simulink subsystem "OpcodeDecoder"  (R2024b)
settings: Solver=VariableStepAuto  StartTime=0.0  StopTime=10.0  RelTol=1e-3
settings Model: Creator=stefano  LastModifiedBy=stefano

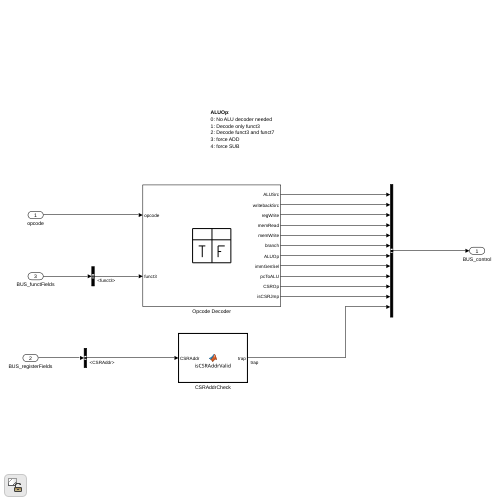
[thumbnail: Simulink's stored preview of the top-level diagram]
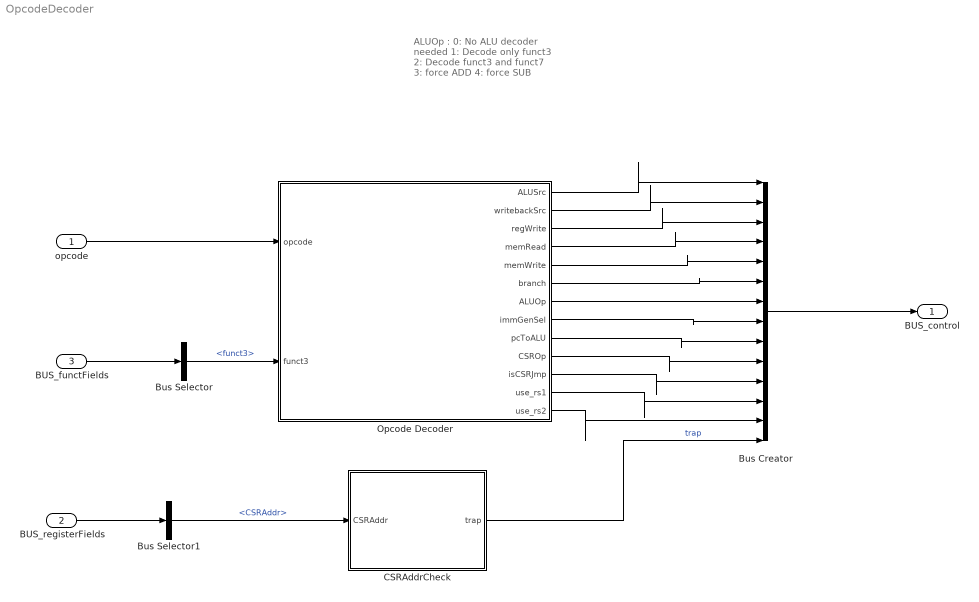
== system OpcodeDecoder ==
  note: ALUOp :
      | 0: No ALU decoder needed
      | 1: Decode only funct3
      | 2: Decode funct3 and funct7
      | 3: force ADD
      | 4: force SUB
  opcode : Inport
  BUS_registerFields : Inport  Port=2
  BUS_functFields : Inport  Port=3
  Bus Creator : BusCreator  Inputs=14
  Bus Selector : BusSelector  OutputSignals=funct3
  Bus Selector1 : BusSelector  OutputSignals=CSRAddr
  CSRAddrCheck : MATLAB Function  TreatAsAtomicUnit=on
  Opcode Decoder : Truth Table  TreatAsAtomicUnit=on
  BUS_control : Outport
  wires:
  Opcode Decoder/5(memWrite) -> Bus Creator/5
  opcode/1 -> Opcode Decoder/1(opcode)
  Opcode Decoder/8(immGenSel) -> Bus Creator/8
  Opcode Decoder/4(memRead) -> Bus Creator/4
  Opcode Decoder/2(writebackSrc) -> Bus Creator/2
  Opcode Decoder/3(regWrite) -> Bus Creator/3
  Bus Creator/1 -> BUS_control/1
  Opcode Decoder/1(ALUSrc) -> Bus Creator/1
  Opcode Decoder/7(ALUOp) -> Bus Creator/7
  Opcode Decoder/9(pcToALU) -> Bus Creator/9
  Opcode Decoder/6(branch) -> Bus Creator/6
  BUS_functFields/1 -> Bus Selector/1
  Bus Selector/1 -> Opcode Decoder/2(funct3)  "<funct3>"
  Opcode Decoder/10(CSROp) -> Bus Creator/10
  CSRAddrCheck/1(trap) -> Bus Creator/14  "trap"
  Bus Selector1/1 -> CSRAddrCheck/1(CSRAddr)  "<CSRAddr>"
  BUS_registerFields/1 -> Bus Selector1/1
  Opcode Decoder/11(isCSRJmp) -> Bus Creator/11
  Opcode Decoder/12(use_rs1) -> Bus Creator/12
  Opcode Decoder/13(use_rs2) -> Bus Creator/13

== matlab function OpcodeDecoder/Opcode Decoder ==
  data: opcode input; ALUSrc output boolean; writebackSrc output fixdt(0,2,0); regWrite output boolean; memRead output boolean; memWrite output boolean; branch output fixdt(0,3,0); ALUOp output fixdt(0,3,0); immGenSel output uint8; pcToALU output boolean; funct3 input; CSROp output boolean; isCSRJmp output boolean; use_rs1 output boolean; use_rs2 output boolean
function [ALUSrc, writebackSrc, regWrite, memRead, memWrite, branch, ALUOp, immGenSel, pcToALU, CSROp, isCSRJmp, use_rs1, use_rs2] = fcn(opcode, funct3)

aVarTruthTableCondition_1 = false;
aVarTruthTableCondition_2 = false;
aVarTruthTableCondition_3 = false;
aVarTruthTableCondition_4 = false;
aVarTruthTableCondition_5 = false;
aVarTruthTableCondition_6 = false;
aVarTruthTableCondition_7 = false;
aVarTruthTableCondition_8 = false;
aVarTruthTableCondition_9 = false;
aVarTruthTableCondition_10 = false;
aVarTruthTableCondition_11 = false;
aVarTruthTableCondition_12 = false;
aVarTruthTableCondition_13 = false;
aVarTruthTableCondition_14 = false;


% R-Type

aVarTruthTableCondition_1 = logical(opcode == 51);

% I-Type - Memory

aVarTruthTableCondition_2 = logical(opcode == 3);

% I-Type - Arithmetical funct3 and funct7

aVarTruthTableCondition_3 = logical(opcode == 19 && (funct3 == 1 || funct3 == 5));

% I-Type - Arithmetical funct3 only

aVarTruthTableCondition_4 = logical(opcode == 19);

% S-Type

aVarTruthTableCondition_5 = logical(opcode == 35);

% SB-Type

aVarTruthTableCondition_6 = logical(opcode == 99);

% U-Type - LUI

aVarTruthTableCondition_7 = logical(opcode == 55);

% U-Type - AUIPC

aVarTruthTableCondition_8 = logical(opcode == 23);

% J-Type - JAL

aVarTruthTableCondition_9 = logical(opcode == 111);

% J-Type - JALR

aVarTruthTableCondition_10 = logical(opcode == 103);

% CSR - ecall

aVarTruthTableCondition_11 = logical(opcode == 115 && funct3 == 0);

% CSR

aVarTruthTableCondition_12 = logical(opcode == 115);

% FENCE

aVarTruthTableCondition_13 = logical(opcode == 15);

% Redirect - NO_OP

aVarTruthTableCondition_14 = logical(opcode == 115);

if (aVarTruthTableCondition_1)
    R();
elseif (aVarTruthTableCondition_2)
    I_mem();
elseif (aVarTruthTableCondition_3)
    I_arithm_3_7();
elseif (aVarTruthTableCondition_4)
    I_arithm_3();
elseif (aVarTruthTableCondition_5)
    S();
elseif (aVarTruthTableCondition_6)
    SB();
elseif (aVarTruthTableCondition_7)
    U_LUI();
elseif (aVarTruthTableCondition_8)
    U_AUIPC();
elseif (aVarTruthTableCondition_9)
    JAL();
elseif (aVarTruthTableCondition_10)
    JALR();
elseif (aVarTruthTableCondition_11)
    CSR_jmp();
elseif (aVarTruthTableCondition_12)
    CSR();
elseif (aVarTruthTableCondition_13)
    NO_OP();
elseif (aVarTruthTableCondition_14)
    NO_OP();
else % Default
    DA();
end

function DA()

% default action (should never reach)

ALUSrc = false;
writebackSrc = 0;
regWrite = false;
memRead = false;
memWrite = false;
branch = 0;
ALUOp = 3;
immGenSel = 0;
pcToALU = false;
CSROp = false;
isCSRJmp = false;
use_rs1 = false;
use_rs2 = false;

function R()

% R-Type

ALUSrc = false;
writebackSrc = 1;
regWrite = true;
memRead = false;
memWrite = false;
branch = 0;
ALUOp = 2;
immGenSel = 0;
pcToALU = false;
CSROp = false;
isCSRJmp = false;
use_rs1 = true;
use_rs2 = true;

function I_mem()

% I-Type - Memory

ALUSrc = true;
writebackSrc = 0;
regWrite = true;
memRead = true;
memWrite = false;
branch = 0;
ALUOp = 3;
immGenSel = 0;
pcToALU = false;
CSROp = false;
isCSRJmp = false;
use_rs1 = true;
use_rs2 = false;

function I_arithm_3()

% I-Type - Arithmetical (funct 3 only)

ALUSrc = true;
writebackSrc = 1;
regWrite = true;
memRead = false;
memWrite = false;
branch = 0;
ALUOp = 1;
immGenSel = 0;
pcToALU = false;
CSROp = false;
isCSRJmp = false;
use_rs1 = true;
use_rs2 = false;

function I_arithm_3_7()

% I-Type - Arithmetical (funct 3 and funct7)

ALUSrc = true;
writebackSrc = 1;
regWrite = true;
memRead = false;
memWrite = false;
branch = 0;
ALUOp = 2;
immGenSel = 0;
pcToALU = false;
CSROp = false;
isCSRJmp = false;
use_rs1 = true;
use_rs2 = false;

function S()

% S -Type

ALUSrc = true;
writebackSrc = 0;
regWrite = false;
memRead = false;
memWrite = true;
branch = 0;
ALUOp = 3;
immGenSel = 1;
pcToALU = false;
CSROp = false;
isCSRJmp = false;
use_rs1 = true;
use_rs2 = true;

function SB()

% SB-Type

ALUSrc = false;
writebackSrc = 0;
regWrite = false;
memRead = false;
memWrite = false;
branch = 1;
ALUOp = 4;
immGenSel = 2;
use_rs1 = true;
use_rs2 = true;
pcToALU = false;
CSROp = false;
isCSRJmp = false;

function U_LUI()

% U-Type - LUI

ALUSrc = true;
writebackSrc = 1;
regWrite = true;
memRead = false;
memWrite = false;
branch = 0;
ALUOp = 0;
immGenSel = 3;
pcToALU = false;
CSROp = false;
use_rs1 = false;
use_rs2 = false;
isCSRJmp = false;

function U_AUIPC()

% U-Type - AUIPC

ALUSrc = true;
writebackSrc = 1;
regWrite = true;
memRead = false;
memWrite = false;
branch = 0;
ALUOp = 3;
immGenSel = 3;
pcToALU = true;
use_rs1 = false;
use_rs2 = false;
CSROp = false;
isCSRJmp = false;

function JAL()

% J-Type - JAL

ALUSrc = true;
writebackSrc = 2;
regWrite = true;
memRead = false;
memWrite = false;
branch = 2;
ALUOp = 3;
immGenSel = 4;
pcToALU = true;
CSROp = false;
isCSRJmp = false;
use_rs1 = false;
use_rs2 = false;

function JALR()

% J-Type - JALR

ALUSrc = true;
writebackSrc = 2;
regWrite = true;
memRead = false;
memWrite = false;
branch = 3;
ALUOp = 3;
immGenSel = 0;
pcToALU = false;
CSROp = false;
isCSRJmp = false;
use_rs1 = false;
use_rs2 = false;

function CSR()

% CSR

ALUSrc = true;
writebackSrc = 2;
regWrite = true;
memRead = false;
memWrite = false;
branch = 0;
ALUOp = 3;
immGenSel = 5;
pcToALU = false;
CSROp = true;
isCSRJmp = false;
use_rs1 = false;
use_rs2 = false;

function CSR_jmp()

% CSR - JMP

ALUSrc = true;
writebackSrc = 2;
regWrite = true;
memRead = false;
memWrite = false;
branch = 4;
ALUOp = 3;
immGenSel = 5;
pcToALU = false;
CSROp = true;
isCSRJmp= true;
use_rs1 = false;
use_rs2 = false;

function NO_OP()

% NO_OP

ALUSrc = true;
writebackSrc = 0;
regWrite = false;
memRead = false;
memWrite = false;
branch = 0;
ALUOp = 0;
immGenSel = 0;
pcToALU = false;
CSROp = false;
isCSRJmp = false;use_rs1 = false;
use_rs2 = false;

== matlab function OpcodeDecoder/CSRAddrCheck ==
  data: CSRAddr input; trap output; valid_csrs parameter size=numel(valid_csrs)
function trap = isCSRAddrValid(CSRAddr, valid_csrs)
%#codegen
trap = true;

for i = 1:length(valid_csrs)
    if CSRAddr == valid_csrs(i)
        trap=false;
        % break;
    end
end
end
